simulink model "calcTangentialCoord_th"  (R2020a)
settings: Solver=VariableStepAuto  StartTime=0.0  StopTime=0  RelTol=1e-3
libraries: calcTangentialCoord_ul x1
settings Model: Creator=Ayaz  LastModifiedBy=Ayaz

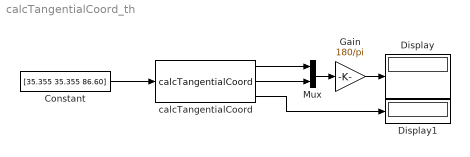
== system calcTangentialCoord_th ==
  Constant : Constant  Value=[35.355 35.355 86.60]
  Display : Display
  Display1 : Display
  Gain : Gain  Gain=180/pi
  Mux : Mux  Inputs=2
  calcTangentialCoord : calcTangentialCoord_ul/calcTangentialCoord  SystemSampleTime=-1  Latency=0  AutoFrameSizeCalculation=off
  wires:
  calcTangentialCoord/1 -> Mux/1
  calcTangentialCoord/2 -> Mux/2
  Constant/1 -> calcTangentialCoord/1
  Mux/1 -> Gain/1
  Gain/1 -> Display/1
  calcTangentialCoord/3 -> Display1/1
